simulink model "Plant3"  (R2016b)
settings: Solver=ode4  StartTime=0.0  StopTime=4000  FixedStep=0.5  RelTol=1e-3  EnableMultiTasking=on
InitFcn:
  | init
libraries: fuzblock x1
settings Model: Creator=Administrator  LastModifiedBy=Truc
settings DataIOCC: LimitDataPoints=on  SaveFormat=Array
settings OptimizationCC: LifeSpan=inf
settings DebuggingCC: UnderspecifiedInitializationDetection=Classic  MergeDetectMultiDrivingBlocksExec=none  SolverPrmCheckMsg=warning  StateNameClashWarn=warning  SFUnexpectedBacktrackingDiag=warning  SFNoUnconditionalDefaultTransitionDiag=warning  SFExecutionAtInitializationDiag=none
settings HardwareCC: ProdBitPerPointer=32  ProdBitPerSizeT=32  ProdBitPerPtrDiffT=32  ProdLargestAtomicFloat=None  ProdIntDivRoundTo=Undefined  ProdEndianess=Unspecified  ProdWordSize=32  ProdHWDeviceType=32-bit Generic
settings ModelReferenceCC: PropagateSignalLabelsOutOfModel=off
settings GRTTargetCC: TargetLangStandard=C89/C90 (ANSI)  GeneratePreprocessorConditionals=Disable all
settings ConfigComp: CovMetricSettings=dw  CovHtmlReporting=on  CovSaveCumulativeToWorkspaceVar=on  CovSaveSingleToWorkspaceVar=on  CovExternalEMLEnable=off

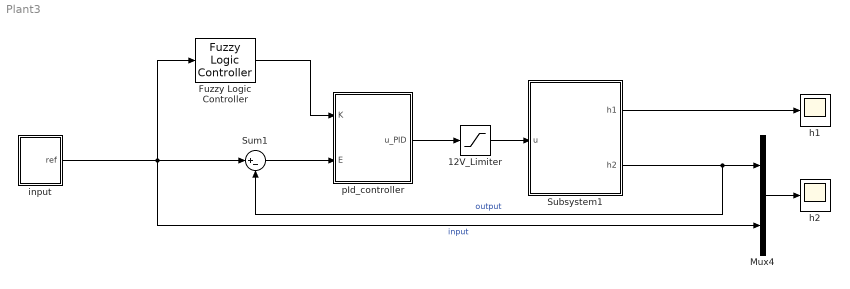
== system Plant3 ==
  12V_Limiter : Saturate  UpperLimit=12  LowerLimit=0
  Fuzzy Logic Controller : fuzblock/Fuzzy Logic  Controller  fis='ObservedPIDFuzzy.fis'
  Mux4 : Mux  Inputs=2
  Subsystem1 : Subsystem  mask{k=4, A_1=9.6211, A_2=9.6211, a1=0.1257, a2=0.0707, g=981}
      mask prompts: k "He so luu luong (k)"; A_1 "Tiet dien bon 1 (A_1)"; A_2 "Tiet dien bon 2 (A_2)"; a1 "Tiet dien van 1 (a1)"; a2 "Tiet dien van 2 (a2)"; g "Trong truong (g)"
  Sum1 : Sum  Inputs=|+-
  h1 : Scope
  h2 : Scope
  input : Subsystem
  pId_controller : Subsystem
  wires:
  Subsystem1/1(h1) -> h1/1
  Subsystem1/2(h2) -> Sum1/2, Mux4/1  "output"
  pId_controller/1(u_PID) -> 12V_Limiter/1
  input/1(ref) -> Sum1/1, Fuzzy Logic Controller/1, Mux4/2  "input"
  Sum1/1 -> pId_controller/2(E)
  Mux4/1 -> h2/1
  Fuzzy Logic Controller/1 -> pId_controller/1(K)
  12V_Limiter/1 -> Subsystem1/1(u)

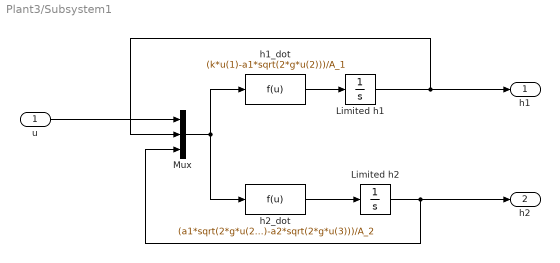
== system Plant3/Subsystem1 ==
  u : Inport
  Limited h1 : Integrator  LimitOutput=on  UpperSaturationLimit=50  LowerSaturationLimit=0
  Limited h2 : Integrator  LimitOutput=on  UpperSaturationLimit=50  LowerSaturationLimit=0
  Mux : Mux  Inputs=3
  h1_dot : Fcn  Expr=(k*u(1)-a1*sqrt(2*g*u(2)))/A_1
  h2_dot : Fcn  Expr=(a1*sqrt(2*g*u(2))-a2*sqrt(2*g*u(3)))/A_2
  h1 : Outport
  h2 : Outport  Port=2
  wires:
  h2_dot/1 -> Limited h2/1
  Limited h2/1 -> h2/1, Mux/3
  Mux/1 -> h2_dot/1, h1_dot/1
  h1_dot/1 -> Limited h1/1
  Limited h1/1 -> h1/1, Mux/2
  u/1 -> Mux/1

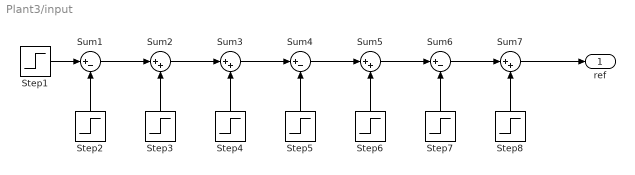
== system Plant3/input ==
  Step1 : Step  Time=0  After=15  SampleTime=0
  Step2 : Step  Time=500  After=10  SampleTime=0
  Step3 : Step  Time=1000  After=5  SampleTime=0
  Step4 : Step  Time=1500  After=10  SampleTime=0
  Step5 : Step  Time=2000  After=10  SampleTime=0
  Step6 : Step  Time=2500  After=15  SampleTime=0
  Step7 : Step  Time=3000  After=5  SampleTime=0
  Step8 : Step  Time=3500  After=15  SampleTime=0
  Sum1 : Sum  Inputs=|+-  SaturateOnIntegerOverflow=on
  Sum{2..3,5,7} (4 alike) : Sum  Inputs=|++  SaturateOnIntegerOverflow=on
  Sum4 : Sum  Inputs=|+-  SaturateOnIntegerOverflow=on
  Sum6 : Sum  Inputs=|+-  SaturateOnIntegerOverflow=on
  ref : Outport
  wires:
  Sum6/1 -> Sum7/1
  Step8/1 -> Sum7/2
  Sum5/1 -> Sum6/1
  Step7/1 -> Sum6/2
  Step6/1 -> Sum5/2
  Sum3/1 -> Sum4/1
  Sum4/1 -> Sum5/1
  Step5/1 -> Sum4/2
  Step4/1 -> Sum3/2
  Sum2/1 -> Sum3/1
  Step3/1 -> Sum2/2
  Sum1/1 -> Sum2/1
  Step1/1 -> Sum1/1
  Step2/1 -> Sum1/2
  Sum7/1 -> ref/1

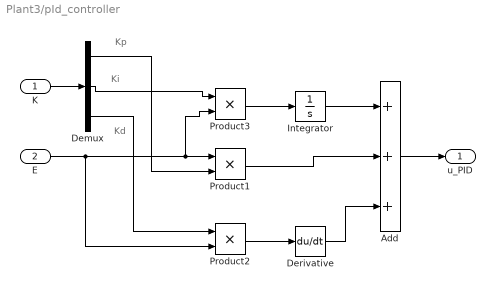
== system Plant3/pId_controller ==
  note: Kp
  note: Ki
  note: Kd
  K : Inport
  E : Inport  Port=2
  Add : Sum  Inputs=+++
  Demux : Demux  Outputs=3
  Derivative : Derivative
  Integrator : Integrator
  Product1 : Product
  Product2 : Product
  Product3 : Product
  u_PID : Outport
  wires:
  Product1/1 -> Add/2
  Demux/1 -> Product1/2
  E/1 -> Product2/2, Product1/1, Product3/2
  Demux/3 -> Product2/1
  Product3/1 -> Integrator/1
  K/1 -> Demux/1
  Integrator/1 -> Add/1
  Product2/1 -> Derivative/1
  Demux/2 -> Product3/1
  Add/1 -> u_PID/1
  Derivative/1 -> Add/3
